simulink model "Arm_Control_Tuning_v001"  (R2017b)
settings: Solver=VariableStepAuto  StartTime=0.0  StopTime=10.0  MaxStep=0.01  RelTol=1e-3
settings Model: Creator=Martin  LastModifiedBy=GEH-Magnet School 1

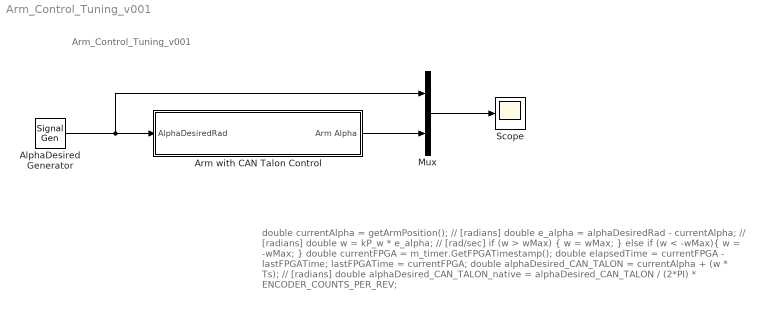
== system Arm_Control_Tuning_v001 ==
  note: double currentAlpha = getArmPosition();						// [radians]
      | double e_alpha = alphaDesiredRad - currentAlpha; 			// [radians]
      | double w = kP_w * e_alpha;									// [rad/sec]
      | if (w > wMax) {		w = wMax;	}	else if (w < -wMax){		w = -wMax;	}
      |
      | double currentFPGA = m_timer.GetFPGATimestamp();
      | double elapsedTime = currentFPGA - lastFPGATime;
      | 	lastFPGATime = currentFPGA;
      | double alphaDesired_CAN_TALON = currentAlpha + (w * Ts);		// [radians]
      | double alphaDesired_CAN_TALON_native = alphaDesired_CAN_TALON / (2*PI) * ENCODER_COUNTS_PER_REV;
  note: Arm_Control_Tuning_v001
  AlphaDesired Generator : SignalGenerator  WaveForm=square  Amplitude=10  Frequency=0.5
  "Arm with CAN Talon Control " : Subsystem
  Mux : Mux  Inputs=2
  Scope : Scope
  wires:
  AlphaDesired Generator/1 -> Mux/1, "Arm with CAN Talon Control "/1(AlphaDesiredRad)
  Mux/1 -> Scope/1
  "Arm with CAN Talon Control "/1(Arm Alpha) -> Mux/2

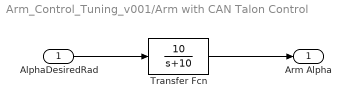
== system Arm_Control_Tuning_v001/Arm with CAN Talon Control  ==
  AlphaDesiredRad : Inport
  Transfer Fcn : TransferFcn  Numerator=10  Denominator=[1 10]
  Arm Alpha : Outport
  wires:
  AlphaDesiredRad/1 -> Transfer Fcn/1
  Transfer Fcn/1 -> Arm Alpha/1
